simulink model "Use_Cases_N3"  (R2020b)
settings: Solver=ode3  StartTime=0.0  StopTime=inf  FixedStep=0.05  RelTol=1e-3
libraries: XBotBlockToolbox x4, simulink x2, Utilities x1

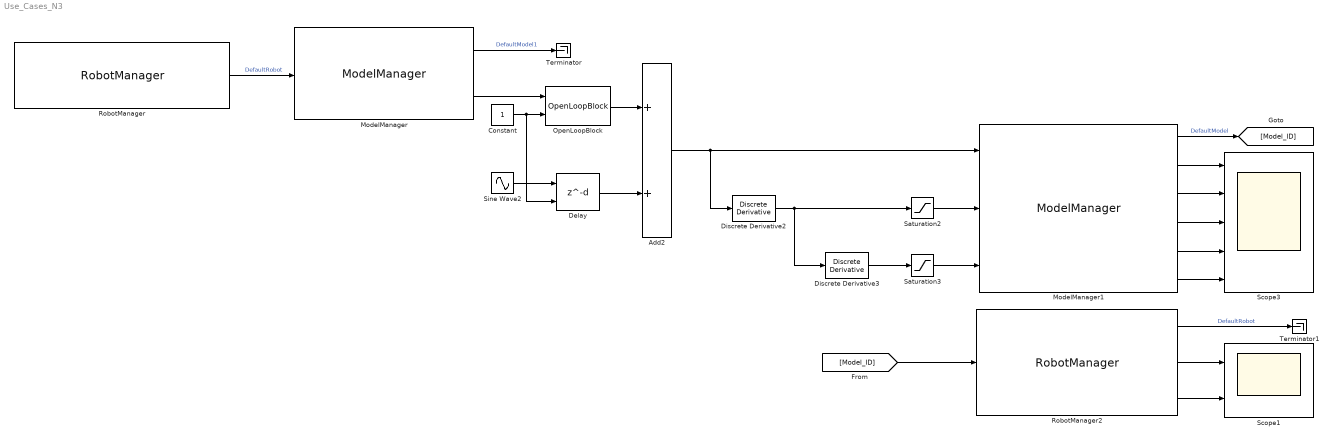
== system Use_Cases_N3 ==
  Add2 : Sum
  Constant : Constant
  Delay : Delay  DelayLengthSource=Input port  DelayLength=1  InitialCondition=0
  Discrete Derivative2 : simulink/Discrete/Discrete Derivative  gainval=1.0  ICPrevScaledInput=0.0  OutMin=[]  OutMax=[]  OutDataType=fixdt(1, 16)  OutScaling=2^-10  DoSatur=off
  Discrete Derivative3 : simulink/Discrete/Discrete Derivative  gainval=1.0  ICPrevScaledInput=0.0  OutMin=[]  OutMax=[]  OutDataType=fixdt(1, 16)  OutScaling=2^-10  DoSatur=off
  ModelManager : XBotBlockToolbox/ModelManager  ModelName=DefaultModel1  RobotName=DefaultRobot  UseExtModel=Off  SyncWithRobot=On  GetFloatingBaseList={}  SetFloatingBaseComponent=Off  GravityRequest=Off  ReadingsList={ 'qJ' }  MechanicalLimitsList={}  MechanicalLimitsCheck=Off  MechanicalLimitsEnforce=Off  SensorList={}  ReferencesList={}  OldModelName=DefaultModel1
  ModelManager1 : XBotBlockToolbox/ModelManager  ModelName=DefaultModel  RobotName=DefaultRobot  UseExtModel=Off  SyncWithRobot=Off  GetFloatingBaseList={}  SetFloatingBaseComponent=Off  GravityRequest=Off  ReadingsList={ 'qJ', 'qJdot', 'qJddot' }  MechanicalLimitsList={}  MechanicalLimitsCheck=On  MechanicalLimitsEnforce=On  SensorList={}  ReferencesList={ 'qJ_ref', 'qJdot_ref', 'qJddot_ref' }  OldModelName=DefaultModel
  OpenLoopBlock : Utilities/OpenLoopBlock  SystemSampleTime=-1  VariantActivationTime=update diagram  Latency=0  AutoFrameSizeCalculation=off
  RobotManager : XBotBlockToolbox/RobotManager  RobotName=DefaultRobot  ModelName=DefaultModel  UseExtRobot=Off  SyncWithModel=Off  ReadingsList={}  MechanicalLimitsList={}  MechanicalLimitsCheck=Off  MechanicalLimitsEnforce=Off  SensorList={}  ReferencesList={}  OldRobotName=DefaultRobot
  RobotManager2 : XBotBlockToolbox/RobotManager  RobotName=DefaultRobot  ModelName=DefaultModel  UseExtRobot=Off  SyncWithModel=On  ReadingsList={ 'qJ', 'qJdot' }  MechanicalLimitsList={}  MechanicalLimitsCheck=Off  MechanicalLimitsEnforce=Off  SensorList={}  ReferencesList={}  OldRobotName=DefaultRobot
  Saturation2 : Saturate  UpperLimit=0.2  LowerLimit=-0.2
  Saturation3 : Saturate  UpperLimit=0.2  LowerLimit=-0.2
  Scope1 : Scope  NumInputPorts=2
  Scope3 : Scope  NumInputPorts=5
  Sine Wave2 : Sin  Amplitude=0.2  SampleTime=0
  Terminator : Terminator
  Terminator1 : Terminator
  wires:
  Add2/1 -> Discrete Derivative2/1, ModelManager1/1
  Sine Wave2/1 -> Delay/1
  Discrete Derivative3/1 -> Saturation3/1
  Saturation3/1 -> ModelManager1/3
  Discrete Derivative2/1 -> Discrete Derivative3/1, Saturation2/1
  ModelManager/2 -> OpenLoopBlock/1
  OpenLoopBlock/1 -> Add2/1
  ModelManager1/2 -> Scope3/1
  ModelManager1/3 -> Scope3/2
  ModelManager1/4 -> Scope3/3
  ModelManager1/1 -> [Model_ID]  "DefaultModel"
  ModelManager/1 -> Terminator/1  "DefaultModel1"
  Saturation2/1 -> ModelManager1/2
  RobotManager/1 -> ModelManager/1  "DefaultRobot"
  RobotManager2/1 -> Terminator1/1  "DefaultRobot"
  [Model_ID] -> RobotManager2/1
  RobotManager2/2 -> Scope1/1
  RobotManager2/3 -> Scope1/2
  Constant/1 -> Delay/2, OpenLoopBlock/2
  ModelManager1/5 -> Scope3/4
  ModelManager1/6 -> Scope3/5
  Delay/1 -> Add2/2
